simulink model "exc2_c"  (R2017a)
settings: Solver=ode45  StartTime=0.0  StopTime=10  RelTol=1e-3  EnableMultiTasking=on
values from neighbouring files (symbols this model uses):
  A = [0 1 0 0;20.6 0 0 0;0 0 0 1;-0.5 0 0 0]    [ask2_A.m]
  B = [0;-1;0;0.5]    [ask2_A.m]
  C = [1 0 0 0;0 0 1 0]    [ask2_A.m]
  initial = [-0.2;-0.06;0.01;0.3]    [ask2_A.m]
  K1 = (ad-a0)*T    [ask2_A.m]
  K3 = K1(3)    [ask2_A.m]
settings Model: Creator=Γιώργος  LastModifiedBy=user
settings DataIOCC: FinalStateName=xFinalc  LimitDataPoints=on  SaveFinalState=on  SaveFormat=Array  SaveState=on  StateSaveName=xoutc  TimeSaveName=toutc  OutputSaveName=youtc  Refine=4
settings OptimizationCC: LifeSpan=inf
settings DebuggingCC: SFUnexpectedBacktrackingDiag=warning  SFNoUnconditionalDefaultTransitionDiag=warning  SFExecutionAtInitializationDiag=none
settings HardwareCC: ProdBitPerPointer=32  ProdBitPerSizeT=32  ProdBitPerPtrDiffT=32  ProdLargestAtomicFloat=None  ProdIntDivRoundTo=Undefined  ProdEndianess=Unspecified  ProdWordSize=32  ProdHWDeviceType=32-bit Generic
settings ModelReferenceCC: PropagateSignalLabelsOutOfModel=off
settings GRTTargetCC: TargetLangStandard=C89/C90 (ANSI)  GeneratePreprocessorConditionals=Disable all
settings ConfigComp: CovMetricSettings=dw  CovHtmlReporting=on  CovSaveCumulativeToWorkspaceVar=on  CovSaveSingleToWorkspaceVar=on  CovExternalEMLEnable=off

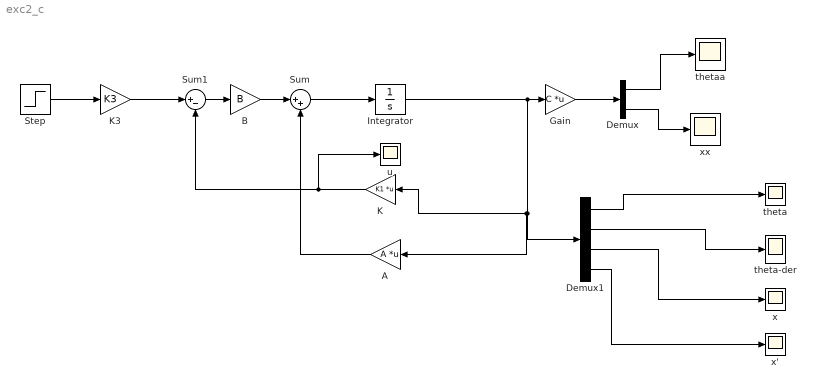
== system exc2_c ==
  A : Gain  Gain=A  Multiplication=Matrix(K*u)
  B : Gain  Gain=B
  Demux : Demux  Outputs=2
  Demux1 : Demux
  Gain : Gain  Gain=C  Multiplication=Matrix(K*u) (u vector)
  Integrator : Integrator  InitialCondition=initial
  K : Gain  Gain=K1  Multiplication=Matrix(K*u)
  K3 : Gain  Gain=K3
  Step : Step  SampleTime=0
  Sum : Sum  Inputs=|++
  Sum1 : Sum  Inputs=|+-
  theta : Scope
  theta-der : Scope
  thetaa : Scope
  u : Scope
  x : Scope
  "x' " : Scope
  xx : Scope
  wires:
  Gain/1 -> Demux/1
  Demux/1 -> thetaa/1
  Demux/2 -> xx/1
  A/1 -> Sum/2
  Sum/1 -> Integrator/1
  K/1 -> Sum1/2, u/1
  Sum1/1 -> B/1
  B/1 -> Sum/1
  Integrator/1 -> Demux1/1, A/1, K/1, Gain/1
  Demux1/1 -> theta/1
  Demux1/2 -> theta-der/1
  Demux1/3 -> x/1
  Demux1/4 -> "x' "/1
  Step/1 -> K3/1
  K3/1 -> Sum1/1
